simulink model "tuningPID"  (R2021b)
settings: Solver=VariableStepAuto  StartTime=0.0  StopTime=1000  RelTol=1e-3
settings Model: Creator=Asus  LastModifiedBy=Asus

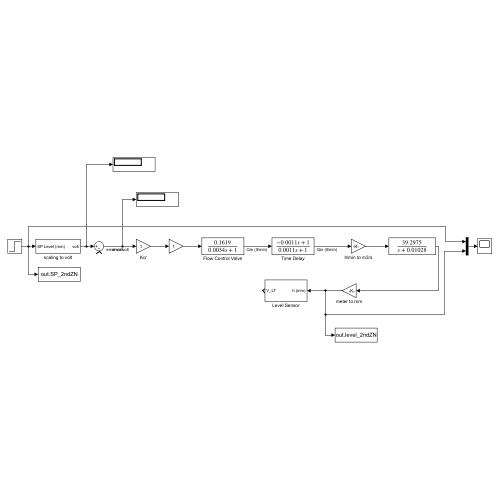
[thumbnail: Simulink's stored preview of the top-level diagram]
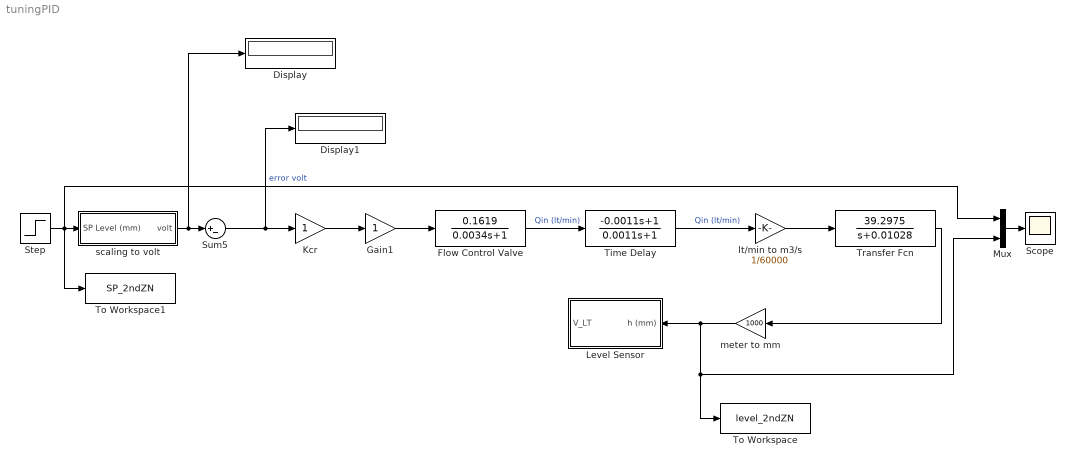
== system tuningPID ==
  Display : Display
  Display1 : Display
  Flow Control Valve : TransferFcn  Numerator=[0.1619]  Denominator=[0.0034 1]
  Gain1 : Gain
  Kcr : Gain
  Level Sensor : Subsystem
  Mux : Mux  Inputs=2
  Scope : Scope
  Step : Step  Time=0  After=100  SampleTime=0
  Sum5 : Sum  Inputs=|+-
  Time Delay : TransferFcn  Numerator=[-0.0011 1]  Denominator=[0.0011 1]
  To Workspace : ToWorkspace  VariableName=level_2ndZN  SampleTime=-1
  To Workspace1 : ToWorkspace  VariableName=SP_2ndZN  SampleTime=-1
  Transfer Fcn : TransferFcn  Numerator=[39.2975]  Denominator=[1 0.01028]
  lt/min to m3/s : Gain  Gain=1/60000
  meter to mm : Gain  Gain=1000
  scaling to volt : Subsystem
  wires:
  scaling to volt/1(volt) -> Display/1, Sum5/1
  Sum5/1 -> Display1/1, Kcr/1  "error volt"
  Flow Control Valve/1 -> Time Delay/1  "Qin (lt/min)"
  Step/1 -> To Workspace1/1, Mux/1, scaling to volt/1(SP Level (mm))
  Time Delay/1 -> lt/min to m3/s/1  "Qin (lt/min)"
  Mux/1 -> Scope/1
  Transfer Fcn/1 -> meter to mm/1
  Kcr/1 -> Gain1/1
  Gain1/1 -> Flow Control Valve/1
  lt/min to m3/s/1 -> Transfer Fcn/1
  meter to mm/1 -> Level Sensor/1(h (mm)), To Workspace/1, Mux/2

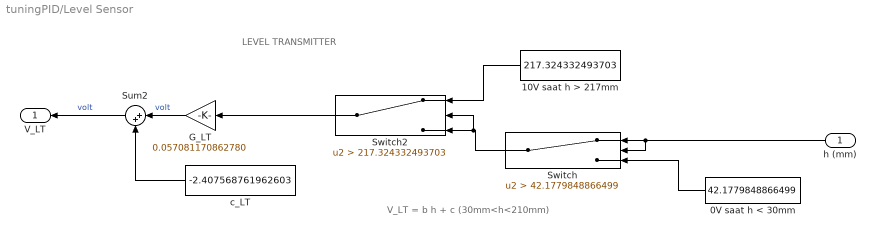
== system tuningPID/Level Sensor ==
  note: V_LT = b h + c (30mm<h<210mm)
  note: LEVEL TRANSMITTER
  h (mm) : Inport
  0V saat h < 30mm : Constant  Value=42.1779848866499
  10V saat h > 217mm : Constant  Value=217.324332493703
  G_LT : Gain  Gain=0.057081170862780
  Sum2 : Sum  Inputs=|++
  Switch : Switch  Criteria=u2 > Threshold  Threshold=42.1779848866499
  Switch2 : Switch  Criteria=u2 > Threshold  Threshold=217.324332493703
  c_LT : Constant  Value=-2.407568761962603
  V_LT : Outport
  wires:
  Switch/1 -> Switch2/2, Switch2/3
  10V saat h > 217mm/1 -> Switch2/1
  G_LT/1 -> Sum2/1  "volt"
  0V saat h < 30mm/1 -> Switch/3
  c_LT/1 -> Sum2/2
  h (mm)/1 -> Switch/2, Switch/1
  Switch2/1 -> G_LT/1
  Sum2/1 -> V_LT/1  "volt"

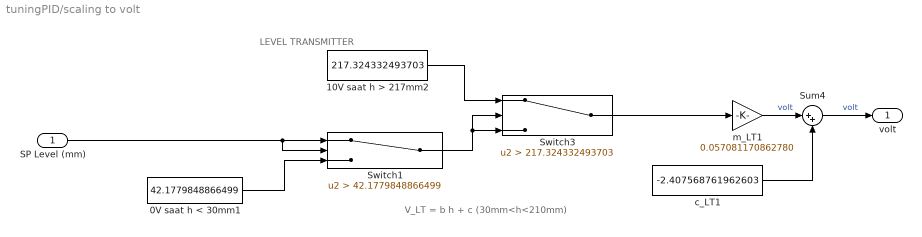
== system tuningPID/scaling to volt ==
  note: LEVEL TRANSMITTER
  note: V_LT = b h + c (30mm<h<210mm)
  SP Level (mm) : Inport
  0V saat h < 30mm1 : Constant  Value=42.1779848866499
  10V saat h > 217mm2 : Constant  Value=217.324332493703
  Sum4 : Sum  Inputs=|++
  Switch1 : Switch  Criteria=u2 > Threshold  Threshold=42.1779848866499
  Switch3 : Switch  Criteria=u2 > Threshold  Threshold=217.324332493703
  c_LT1 : Constant  Value=-2.407568761962603
  m_LT1 : Gain  Gain=0.057081170862780
  volt : Outport
  wires:
  Switch1/1 -> Switch3/2, Switch3/3
  SP Level (mm)/1 -> Switch1/1, Switch1/2
  10V saat h > 217mm2/1 -> Switch3/1
  0V saat h < 30mm1/1 -> Switch1/3
  m_LT1/1 -> Sum4/1  "volt"
  Switch3/1 -> m_LT1/1
  c_LT1/1 -> Sum4/2
  Sum4/1 -> volt/1  "volt"
